simulink model "premiere_ordre_zero"  (R2021b)
settings: Solver=VariableStepAuto  StartTime=0.0  StopTime=10.0  RelTol=1e-3
undefined symbols (not defined in the file): H_1z
libraries: cstblocks x3
settings Model: Creator=sarmeegan  LastModifiedBy=sarmeegan

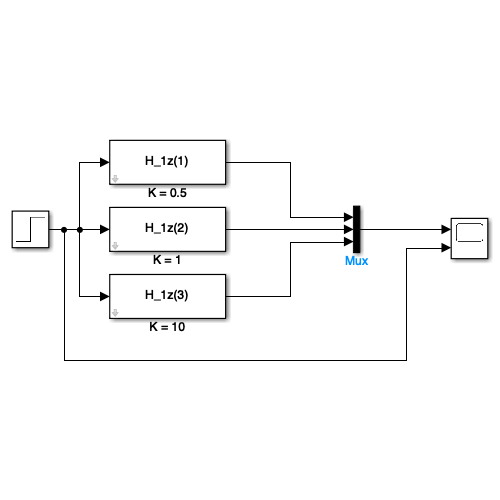
[thumbnail: Simulink's stored preview of the top-level diagram]
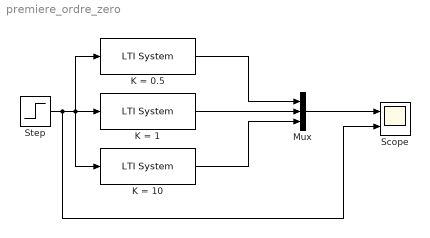
== system premiere_ordre_zero ==
  K = 0.5 : cstblocks/LTI System  sys=H_1z(1)  IC=[]
  K = 1 : cstblocks/LTI System  sys=H_1z(2)  IC=[]
  K = 10 : cstblocks/LTI System  sys=H_1z(3)  IC=[]
  Mux : Mux  Inputs=3
  Scope : Scope  NumInputPorts=2
  Step : Step  Time=0  SampleTime=0
  wires:
  Step/1 -> Scope/2, K = 10/1, K = 0.5/1, K = 1/1
  K = 0.5/1 -> Mux/1
  K = 1/1 -> Mux/2
  K = 10/1 -> Mux/3
  Mux/1 -> Scope/1
